simulink model "BBB_USRLED_Test"  (R2013a)
settings: Solver=FixedStepDiscrete  SolverMode=SingleTasking  StartTime=0.0  StopTime=inf  FixedStep=0.001  RelTol=1e-3
libraries: simulink x2
settings Model: SimulationMode=external  ExtModeTrigDuration=100  Creator=rdustinkahawita  LastModifiedBy=rdustinkahawita
settings DataIOCC: InspectSignalLogs=on
settings OptimizationCC: OptimizeModelRefInitCode=on  LifeSpan=1
settings DebuggingCC: SolverPrmCheckMsg=none  StrictBusMsg=Warning
settings HardwareCC: ProdLargestAtomicInteger=Long  ProdLargestAtomicFloat=Double  ProdEndianess=LittleEndian  ProdHWDeviceType=ARM Compatible->ARM Cortex
settings RTWCC: SystemTargetFile=realtime.tlc  GenerateMakefile=off  TemplateMakefile=realtime.tmf  Description=Run on Target Hardware  RTWVerbose=off  ProcessScript=realtime_make_rtw_hook
settings STFCustomTargetCC: TargetLibSuffix=.a  GenerateSampleERTMain=on  ERTCustomFileBanners=on  SupportNonInlinedSFcns=off  SupportVariableSizeSignals=on  MATLABClassNameForMDSCustomization=Simulink.SoftwareTarget.ERTCustomization  SystemTargetFile=realtime.tlc
settings ERTTargetCC: ParMdlRefBuildCompliant=off  CompOptLevelCompliant=off  ConcurrentExecutionCompliant=off  CombineOutputUpdateFcns=off  ERTFirstTimeCompliant=off  SupportContinuousTime=on  SupportVariableSizeSignals=on  ModelStepFunctionPrototypeControlCompliant=off  CPPClassGenCompliant=off  ExtMode=on  ExtModeMexArgs='192.168.7.2' 0 17725  ERTSrcFileBannerTemplate=realtime_code_template.cgt  ERTHdrFileBannerTemplate=realtime_code_template.cgt  ERTDataSrcFileTemplate=realtime_code_template.cgt  ERTDataHdrFileTemplate=realtime_code_template.cgt  ERTCustomFileTemplate=realtime_file_process.tlc

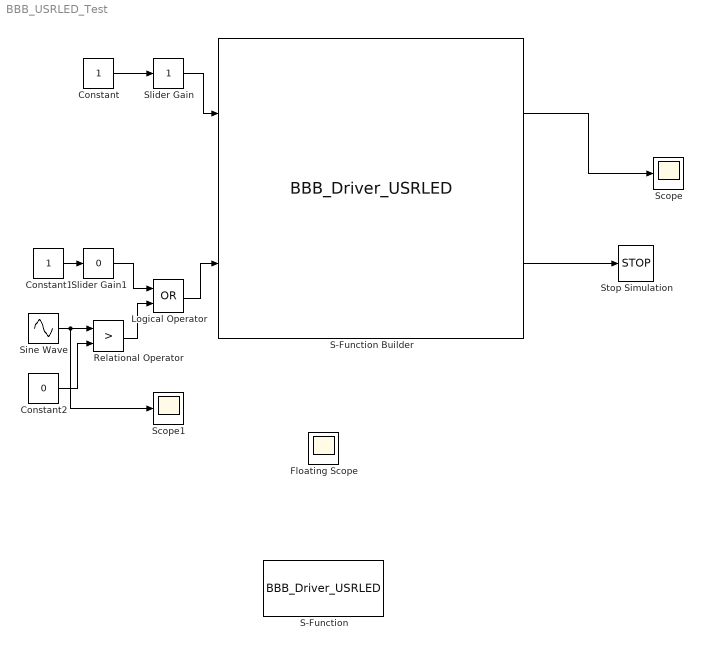
== system BBB_USRLED_Test ==
  Constant : Constant  OutMin=0  OutMax=1  OutDataTypeStr=boolean  LockScale=on
  Constant1 : Constant  OutMin=0  OutMax=1  OutDataTypeStr=boolean  LockScale=on
  Constant2 : Constant  Value=0  OutMin=0  OutMax=1  OutDataTypeStr=boolean  LockScale=on
  Floating Scope : Scope
      settings: Floating=on  SaveName=ScopeData2
  Logical Operator : Logic  Operator=OR  AllPortsSameDT=off  OutDataTypeStr=boolean
  Relational Operator : RelationalOperator  Operator=>  OutDataTypeStr=boolean
  S-Function : S-Function  FunctionName=BBB_Driver_USRLED  Parameters=uint8(4),uint8(6)  SFunctionModules=BBB_Driver_USRLED_wrapper  EnableBusSupport=off
  S-Function Builder : S-Function  InitFcn=try, set_param(gcb,'FunctionName','BBB_Driver_USRLED'), end  FunctionName=BBB_Driver_USRLED  Parameters=uint8(4),uint8(6)  SFunctionModules=BBB_Driver_USRLED_wrapper  EnableBusSupport=off  mask(S-Function Builder){}
      mask help: Simulink:masks:SFunctionBuilder_MD
      mask init:
      | val = [[.9  0.75 0.75 1 1 .9 .9 1]',[1 1 0.75 0.75 .9 .9 1 .9]'];try , sys = get_param(gcb,'SfunBuilderFcnName');if isempty(sys), sys = get_param(gcb,'FunctionName'); end,catch, sys = get_param(gcb,'FunctionName'); end
      settings: CopyFcn=set_param(gcbh,'LinkStatus','none')  PreSaveFcn=try, set_param(gcb,'FunctionName','BBB_Driver_USRLED'), end  OpenFcn=sfunctionwizard(gcbh)
      mask Display: plot(val(:,1),val(:,2)),disp(sys), port_label('input',1,'inUSRLED_Enable'), port_label('input',2,'inUSRLED_On_Trigger'), port_label('output',1,'outUSRLED_State'), port_label('output',2,'outSimStop')
  Scope : Scope
      settings: TimeRange=10
  Scope1 : Scope
      settings: TimeRange=10
  Sine Wave : Sin  Frequency=5
  Slider Gain : simulink/Math Operations/Slider Gain  low=0  gain=1  high=1
  Slider Gain1 : simulink/Math Operations/Slider Gain  low=0  gain=0  high=1
  Stop Simulation : Stop
  wires:
  Constant/1 -> Slider Gain/1
  S-Function Builder/1 -> Scope/1
  Slider Gain/1 -> S-Function Builder/1
  Constant1/1 -> Slider Gain1/1
  S-Function Builder/2 -> Stop Simulation/1
  Slider Gain1/1 -> Logical Operator/1
  Constant2/1 -> Relational Operator/2
  Sine Wave/1 -> Scope1/1, Relational Operator/1
  Relational Operator/1 -> Logical Operator/2
  Logical Operator/1 -> S-Function Builder/2
